simulink model "system_dyninv_olp"  (R2018b)
settings: Solver=ode8  StartTime=0.0  StopTime=10  FixedStep=0.01  RelTol=1e-3
values from neighbouring files (symbols this model uses):
  A = [0 1; -w^2 -2*z*w]    [dyninv_2nd_order.m]
  B = [0; w^2]    [dyninv_2nd_order.m]
  C = [1 0; 0 1]    [dyninv_2nd_order.m]
settings Model: Creator=suvo.ganguli  LastModifiedBy=suvo.ganguli

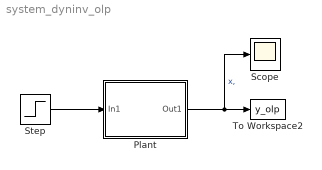
== system system_dyninv_olp ==
  Plant : Subsystem
  Scope : Scope
  Step : Step  SampleTime=0
  To Workspace2 : ToWorkspace  VariableName=y_olp  SampleTime=-1
  wires:
  Plant/1(Out1) -> To Workspace2/1, Scope/1  "x,"
  Step/1 -> Plant/1(In1)

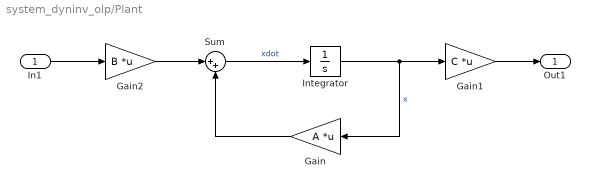
== system system_dyninv_olp/Plant ==
  In1 : Inport
  Gain : Gain  Gain=A  Multiplication=Matrix(K*u)
  Gain1 : Gain  Gain=C  Multiplication=Matrix(K*u)
  Gain2 : Gain  Gain=B  Multiplication=Matrix(K*u)
  Integrator : Integrator
  Sum : Sum  Inputs=|++
  Out1 : Outport
  wires:
  Integrator/1 -> Gain1/1, Gain/1  "x"
  Sum/1 -> Integrator/1  "xdot"
  Gain/1 -> Sum/2
  In1/1 -> Gain2/1
  Gain2/1 -> Sum/1
  Gain1/1 -> Out1/1
